simulink model "smm_gait_control"  (R2018b)
settings: configuration reference "Configuration1khz" (kept outside this file)
InitFcn:
  | addpath('./functions/')
  | addpath('./policies/')
  | control_params
values from neighbouring files (symbols this model uses):
  rest = extract_policy_variables('policies/rest.mat')    [control_params.m]
  run_slow = extract_policy_variables('policies/06_run_reduced.mat')    [control_params.m]
  walk_slow = extract_policy_variables('policies/06_walk.mat')    [control_params.m]
undefined symbols (not defined in the file or in its folder): ctrl, Discrete, initial_dx_estimate, initial_dy_estimate, initial_dz_estimate, initial_z_estimate, sample_time, Time
libraries: simulink x42, ctrlSharedLib x7
(part 4 of 5)

== system smm_gait_control/Behavior/Swing Leg Control Secondary/Back//Front PD (velocity) ==
  Desired Position [rad] [back front] : Inport
  Desired Velocity [rad/s] [back front] : Inport  Port=2
  Desired Acceleration [rad/s^2] [back front] : Inport  Port=3
  Measured Position [rad] [back front] : Inport  Port=4
  Measured Velocity [rad/s] [back front] : Inport  Port=5
  Back / Front PositionTracking : Scope  NumInputPorts=2
  Back / Front Velocity Tracking : Scope  NumInputPorts=2
  Feedback / Feedforward : Scope  NumInputPorts=2
  Feedforward Gain : Gain
  Kp_SEA_Trajectory : Constant  Value=ctrl.kp_velocity_swing
  Mux{1..2,12..13} (4 alike) : Mux  Inputs=2
  Product1 : Product
  Selector{,1..3} (4 alike) : Selector  InputPortWidth=2  IndexOptions=Index vector (dialog)  Indices=[1]  OutputSizes=1
  Selector{4..5,7..8} (4 alike) : Selector  InputPortWidth=2  IndexOptions=Index vector (dialog)  Indices=[2]  OutputSizes=1
  Sum7 : Sum  Inputs=|+-
  Sum9 : Sum
  Terminator : Terminator
  Commanded Velocity [rad/s] [back front] : Outport
  wires:
  Kp_SEA_Trajectory/1 -> Product1/2
  Sum9/1 -> Commanded Velocity [rad/s] [back front]/1
  Measured Position [rad] [back front]/1 -> Selector4/1, Selector/1, Sum7/2
  Sum7/1 -> Product1/1
  Product1/1 -> Feedback / Feedforward/1, Sum9/1
  Mux13/1 -> Back / Front PositionTracking/1
  Desired Position [rad] [back front]/1 -> Selector5/1, Selector1/1, Sum7/1
  Mux2/1 -> Back / Front PositionTracking/2
  Selector/1 -> Mux13/1
  Selector1/1 -> Mux13/2
  Selector5/1 -> Mux2/2
  Selector4/1 -> Mux2/1
  Desired Velocity [rad/s] [back front]/1 -> Feedforward Gain/1, Selector8/1, Selector3/1
  Feedforward Gain/1 -> Feedback / Feedforward/2, Sum9/2
  Desired Acceleration [rad/s^2] [back front]/1 -> Terminator/1
  Measured Velocity [rad/s] [back front]/1 -> Selector7/1, Selector2/1
  Mux1/1 -> Back / Front Velocity Tracking/1
  Selector2/1 -> Mux1/1
  Selector7/1 -> Mux12/1
  Mux12/1 -> Back / Front Velocity Tracking/2
  Selector8/1 -> Mux12/2
  Selector3/1 -> Mux1/2

== system smm_gait_control/Behavior/Swing Leg Control Secondary/Lateral PD (torque) ==
  note: (Approximation)
      | This is the lateral torque generated due to the relative
      | acceleration of the motor around the pelvis. Only
      | approximate vertical components are used in the
      | calculation. The lateral components are small.
  Desired Position [rad] : Inport
  Desired Velocity [rad/s] : Inport  Port=2
  Desired Acceleration [rad/s^2] : Inport  Port=3
  Measured Position [rad] : Inport  Port=4
  Measured Velocity [rad/s] : Inport  Port=5
  CoM Z Acceleration [m/s^2] : Inport  Port=6
  Feedback / Feedforward : Scope  NumInputPorts=2
  Kp_SEA_Trajectory : Constant  Value=ctrl.kp_lateral_swing
  Kp_SEA_Trajectory1 : Constant  Value=ctrl.kd_lateral_swing
  Kp_SEA_Trajectory2 : Constant  Value=ctrl.i_lateral_about_pelvis
  Kp_SEA_Trajectory3 : Constant  Value=ctrl.lateral_offset
  Kp_SEA_Trajectory4 : Constant  Value=(ctrl.m_leg_motor + ctrl.m_leg)
  Kp_SEA_Trajectory5 : Constant  Value=-ctrl.g
  Mux13 : Mux  Inputs=2
  Mux2 : Mux  Inputs=2
  Position / Velocity Tracking : Scope  NumInputPorts=2
  Product1 : Product
  Product2 : Product
  Product3 : Product
  Product4 : Product  Inputs=3
  Sum1 : Sum  Inputs=|+-
  Sum2 : Sum  Inputs=|++
  Sum3 : Sum  Inputs=|++
  Sum4 : Sum  Inputs=|+-
  Sum7 : Sum  Inputs=|+-
  Sum9 : Sum  Inputs=++|
  Commanded Torque [Nm] : Outport
  wires:
  Sum3/1 -> Sum2/2, Feedback / Feedforward/2
  Kp_SEA_Trajectory2/1 -> Product3/1
  Desired Acceleration [rad/s^2]/1 -> Product3/2
  Sum2/1 -> Commanded Torque [Nm]/1
  Sum9/1 -> Sum2/1, Feedback / Feedforward/1
  Kp_SEA_Trajectory1/1 -> Product2/2
  Sum1/1 -> Product2/1
  Kp_SEA_Trajectory/1 -> Product1/2
  Measured Position [rad]/1 -> Mux13/1, Sum7/2
  Sum7/1 -> Product1/1
  Product1/1 -> Sum9/1
  Mux13/1 -> Position / Velocity Tracking/1
  Desired Position [rad]/1 -> Mux13/2, Sum7/1
  Mux2/1 -> Position / Velocity Tracking/2
  Desired Velocity [rad/s]/1 -> Mux2/2, Sum1/1
  Product2/1 -> Sum9/2
  Measured Velocity [rad/s]/1 -> Mux2/1, Sum1/2
  Product3/1 -> Sum3/1
  Product4/1 -> Sum3/2
  Kp_SEA_Trajectory4/1 -> Product4/3
  Kp_SEA_Trajectory3/1 -> Product4/2
  Kp_SEA_Trajectory5/1 -> Sum4/1
  CoM Z Acceleration [m/s^2]/1 -> Sum4/2
  Sum4/1 -> Product4/1

== system smm_gait_control/Behavior/Tranform Sensor Measurements to CoM Acceleration Measurement/Compute Body Frame Accelerations ==
  imu accelerations x3 : Inport
  IMU Accel Unfiltered vs Filtered : Scope  NumInputPorts=3
  IMU Two Pole Filter2 : DiscreteTransferFcn  Numerator=[ctrl.A_lpf_accelerometer 0 0]  Denominator=[1 ctrl.B1_lpf_accelerometer ctrl.B2_lpf_accelerometer]  SampleTime=sample_time
  Mux : Mux  Inputs=2
  Selector : Selector  InputPortWidth=6  IndexOptions=Index vector (dialog)  Indices=[1 4]  OutputSizes=1
  Selector1 : Selector  InputPortWidth=6  IndexOptions=Index vector (dialog)  Indices=[2 5]  OutputSizes=1
  Selector2 : Selector  InputPortWidth=6  IndexOptions=Index vector (dialog)  Indices=[3 6]  OutputSizes=1
  accelerations [m/s^2] x3 : Outport
  wires:
  Mux/1 -> Selector/1, Selector2/1, Selector1/1
  imu accelerations x3/1 -> IMU Two Pole Filter2/1, Mux/1
  Selector/1 -> IMU Accel Unfiltered vs Filtered/1
  Selector1/1 -> IMU Accel Unfiltered vs Filtered/2
  Selector2/1 -> IMU Accel Unfiltered vs Filtered/3
  IMU Two Pole Filter2/1 -> Mux/2, accelerations [m/s^2] x3/1

== system smm_gait_control/Behavior/Tranform Sensor Measurements to CoM Acceleration Measurement/Estimate Angular Accelerations2 ==
  Angular Velocities [rad/s] x3 : Inport
  Enabled : Inport  Port=2
  Detect Change : simulink/Logic and Bit Operations/Detect Change  vinit=0  OutDataTypeStr=boolean
  Difference : simulink/Discrete/Difference  ICPrevInput=0.0  OutMin=[]  OutMax=[]  OutDataType=fixdt(1, 16)  OutScaling=2^-10  DoSatur=off
  Gain : Gain  Gain=1/sample_time
  IMU Two Pole Filter : DiscreteTransferFcn  Numerator=[ctrl.A_imu 0 0]  Denominator=[1 ctrl.B1_imu ctrl.B2_imu]  SampleTime=sample_time
  Logical Operator5 : Logic  Operator=NOT  AllPortsSameDT=off  OutDataTypeStr=boolean
  Product : Product
  Angular Accelerations [rad/s^2] x3 : Outport
  wires:
  Detect Change/1 -> Logical Operator5/1
  Difference/1 -> Gain/1
  Gain/1 -> Product/1
  Angular Velocities [rad/s] x3/1 -> Difference/1
  Logical Operator5/1 -> Product/2
  Enabled/1 -> Detect Change/1
  Product/1 -> IMU Two Pole Filter/1
  IMU Two Pole Filter/1 -> Angular Accelerations [rad/s^2] x3/1

== system smm_gait_control/Behavior/Tranform Sensor Measurements to CoM Acceleration Measurement/Estimate Angular Accelerations3 ==
  Angular Velocities [rad/s] x2 : Inport
  Enabled : Inport  Port=2
  Detect Change : simulink/Logic and Bit Operations/Detect Change  vinit=0  OutDataTypeStr=boolean
  Difference : simulink/Discrete/Difference  ICPrevInput=0.0  OutMin=[]  OutMax=[]  OutDataType=fixdt(1, 16)  OutScaling=2^-10  DoSatur=off
  Gain : Gain  Gain=1/sample_time
  IMU Two Pole Filter : DiscreteTransferFcn  Numerator=[ctrl.A_lpf_lateral_accel 0 0]  Denominator=[1 ctrl.B1_lpf_lateral_accel ctrl.B2_lpf_lateral_accel]  SampleTime=sample_time
  Logical Operator5 : Logic  Operator=NOT  AllPortsSameDT=off  OutDataTypeStr=boolean
  Product : Product
  Angular Accelerations [rad/s^2] x2 : Outport
  wires:
  Enabled/1 -> Detect Change/1
  Logical Operator5/1 -> Product/2
  Angular Velocities [rad/s] x2/1 -> Difference/1
  Gain/1 -> Product/1
  Difference/1 -> Gain/1
  Detect Change/1 -> Logical Operator5/1
  Product/1 -> IMU Two Pole Filter/1
  IMU Two Pole Filter/1 -> Angular Accelerations [rad/s^2] x2/1

== system smm_gait_control/Behavior/Filtering/Kalman Filtering/Subsystem ==
  right : Inport
  right? : Inport  Port=2
  left : Inport  Port=3
  Switch : Switch  Criteria=u2 ~= 0
  out : Outport
  wires:
  right/1 -> Switch/1
  right?/1 -> Switch/2
  left/1 -> Switch/3
  Switch/1 -> out/1

== system smm_gait_control/Behavior/Filtering/Kalman Filtering/Subsystem1 ==
  right : Inport
  right? : Inport  Port=2
  left : Inport  Port=3
  Switch : Switch  Criteria=u2 ~= 0
  out : Outport
  wires:
  right/1 -> Switch/1
  right?/1 -> Switch/2
  left/1 -> Switch/3
  Switch/1 -> out/1

== system smm_gait_control/Behavior/Filtering/Kalman Filtering/Subsystem2 ==
  right : Inport
  right? : Inport  Port=2
  left : Inport  Port=3
  Switch : Switch  Criteria=u2 ~= 0
  out : Outport
  wires:
  right/1 -> Switch/1
  right?/1 -> Switch/2
  left/1 -> Switch/3
  Switch/1 -> out/1

== system smm_gait_control/Behavior/Motion Planner/Motion Plan with Simplified Model/Toggle Section Number ==
  1 : Inport
  2 : Inport  Port=2
  3 : Inport  Port=3
  Enable : EnablePort
  Cast : DataTypeConversion  OutDataTypeStr=uint8
  Cast1 : DataTypeConversion  OutDataTypeStr=uint8
  Cast2 : DataTypeConversion  OutDataTypeStr=uint8
  Gain : Gain
  Gain1 : Gain  Gain=2
  Gain2 : Gain  Gain=3
  Max : MinMax  Function=max  Inputs=3
  Out : Outport  InitialOutput=1
  wires:
  Gain/1 -> Cast/1
  Gain1/1 -> Cast1/1
  Gain2/1 -> Cast2/1
  Max/1 -> Out/1
  1/1 -> Gain/1
  2/1 -> Gain1/1
  3/1 -> Gain2/1
  Cast1/1 -> Max/2
  Cast2/1 -> Max/3
  Cast/1 -> Max/1

== matlab function smm_gait_control/Behavior/Swing Leg Control Secondary/Avoid Hitting Mechanical Limits ==
  data: back_cmd output double; front_cmd output double; dback_cmd output double; dfront_cmd output double; ddback_cmd output double; ddfront_cmd output double; back_desired input; dback_desired input; ddback_desired input; front_desired input; dfront_desired input; ddfront_desired input; ctrl parameter
%% Avoid fourbar limits by saturating the commands and ensuring we don't command velocities or 
% accelerations that would push us into the limits when nearby
function [back_cmd, front_cmd, dback_cmd, dfront_cmd, ddback_cmd, ddfront_cmd] ...
    = AvoidFourbarLimits(back_desired,dback_desired, ddback_desired, ...
          front_desired, dfront_desired, ddfront_desired, ...
          ctrl)
    [back_cmd, front_cmd, dback_cmd, dfront_cmd, ddback_cmd, ddfront_cmd] = ...
      AvoidFourbarLimits(back_desired, dback_desired, ddback_desired, ...
                         front_desired, dfront_desired, ddfront_desired, ...
                         ctrl.min_front_bar_angle, ctrl.max_front_bar_angle, ...
                         ctrl.min_back_bar_angle, ctrl.max_back_bar_angle);
end

== matlab function smm_gait_control/Behavior/Select Gait Number ==
  data: system_time input; gait_id output; step_number input; enable_locomotion output; at_rest input; disable_locomotion output
function [gait_id, enable_locomotion, disable_locomotion] = select_gait(system_time, step_number, at_rest)

  if system_time < 5
    gait_id = 1;
    enable_locomotion = false;
    disable_locomotion = true;
  else
    enable_locomotion = true;
    disable_locomotion = false;
    if step_number <= 10
      gait_id = 2;
    elseif step_number > 10 && step_number <= 20
      gait_id = 3;
    elseif step_number > 20 && step_number <= 30
      gait_id = 4;
    elseif step_number > 30 && step_number <= 40
      gait_id = 3;
    elseif step_number > 40 && step_number <= 50
      gait_id = 2;
    else
      gait_id = 1;
      if at_rest
        enable_locomotion = false;
        disable_locomotion = true;
      end
    end
  end
      
end

== matlab function smm_gait_control/Behavior/2D Lateral Stance Control2 ==
  data: F_leg input; lateral_torque output; ctrl parameter
function lateral_torque = lateral_stance_control_on_boom(F_leg,ctrl)
    lateral_torque = F_leg*ctrl.lateral_offset*(ctrl.m_total-(ctrl.m_leg_motor+ctrl.m_leg))/ctrl.m_total;
end

== stateflow chart smm_gait_control/Behavior/Contact State Machine/Left Leg State ==
  state Stance
  state Twilight
  state Swing
  (junction 196) -> Stance
  (junction 198) -> (junction 196)
  Stance -> Twilight : [terminate_contact && force < touchdown_threshold]
  Twilight -> Swing : after(ctrl.twilight_time, sec)
  (default) -> Swing
  Swing -> (junction 198) : [force > touchdown_threshold]
  data: force input; touchdown_threshold input; ctrl parameter; Stance output boolean; Twilight output boolean; Swing output boolean; terminate_contact input

== matlab function smm_gait_control/Behavior/2D Lateral Stance Control3 ==
  data: F_leg input; lateral_torque output; ctrl parameter
function lateral_torque = lateral_stance_control_on_boom(F_leg,ctrl)
    lateral_torque = F_leg*ctrl.lateral_offset*(ctrl.m_total-(ctrl.m_leg_motor+ctrl.m_leg))/ctrl.m_total;
end

== matlab function smm_gait_control/Behavior/Centroidal Model Control/Stance Control ==
  data: enable input; x_state_desired output; z_state_desired output; feedforward_term_1 output; feedforward_term_2 output; feedforward_term_3 output; feedback_term_1 output; feedback_term_2 output; feedback_term_3 output; reference input size=[6 1]; K_lqr input size=[3 6]; feedforward_terms input size=[3 1]; phase input; x_state_1 input; x_state_2 input; Fx1 output; z_state input; theta_state input; leg_length_primary input; leg_length_secondary input; Fz_disturbance input; right_is_primary input; plan_not_ready input; Fz1 output; Fx2 output; Fz2 output; ctrl parameter
%% Create motion plans for the centroidal model
% state = [x, dx/dt, z, dz/dt, theta, dtheta/dt]
% F_single_support = [Fx, Fz]
% F_double_support = [Fx, Fz1, Fz2]
function [ x_state_desired, z_state_desired, ...
           feedforward_term_1, feedforward_term_2, feedforward_term_3, ...
           feedback_term_1, feedback_term_2, feedback_term_3, ...
           Fx1, Fz1, Fx2, Fz2] = ...
           centroidal_control(enable, reference, K_lqr, feedforward_terms, ...
                              phase, x_state_1, x_state_2, z_state, theta_state, ...
                              leg_length_primary, leg_length_secondary, Fz_disturbance, right_is_primary, plan_not_ready, ctrl)

  persistent p_prev_x_state_desired p_prev_z_state_desired p_prev_fx1 p_prev_fx2 p_prev_fz1 p_prev_fz2
  if isempty(p_prev_x_state_desired)
    p_prev_x_state_desired = [0; 0]; 
    p_prev_z_state_desired = [0; 0];
    p_prev_fx1 = 0;
    p_prev_fx2 = 0; 
    p_prev_fz1 = 0; 
    p_prev_fz2 = 0;
  end
                            
  % Nothing to be done for flight phase, return
  if phase == 0
    Fx1 = 0;
    Fz1 = 0;
    Fx2 = 0;
    Fz2 = 0;
    x_state_desired = [0; 0];
    z_state_desired = [0; 0];
    feedforward_term_1 = 0;
    feedforward_term_2 = 0;
    feedforward_term_3 = 0;
    feedback_term_1 = 0;
    feedback_term_2 = 0;
    feedback_term_3 = 0;
    p_prev_x_state_desired = [0; 0]; 
    p_prev_z_state_desired = [0; 0];
    p_prev_fx1 = 0;
    p_prev_fx2 = 0; 
    p_prev_fz1 = 0; 
    p_prev_fz2 = 0;
    return;
  end
  
  % Compute feedback control
  error = reference - [x_state_1; z_state; theta_state];
  F_feedback = K_lqr*error;
%   % use neutral feedforward in single support
%   if phase == 1
%     feedforward_terms(2) = acos(min(max(x_state_1(1)/z_state(1),-1),1));
%   end
  % Create control output variables
  input = F_feedback + feedforward_terms; % [Fx, Fz1, Fz2]
  if phase == 1
    F_mag = input(1);
    F_angle = input(2);
    Fx1 = F_mag*cos(F_angle);
    Fz1 = F_mag*sin(F_angle);
    Fz1 = max(Fz1 + Fz_disturbance, 0); % Fz > 0 constraint
    Fz2 = 0;
    Fx1 = max(min(Fx1, 0.5*Fz1), -0.5*Fz1); % saturate to friction cone
    Fx2 = 0;
  else % phase == 2, double support
    Fz1 = input(2);
    Fz2 = input(3);
    Fz1 = max(Fz1 + Fz_disturbance*Fz1/(Fz1+Fz2+eps),0); % Fz > 0 constraint
    Fz2 = max(Fz2 + Fz_disturbance*Fz2/(Fz1+Fz2+eps),0);
    Fx1 = input(1)*Fz1/(Fz1+Fz2+eps); % distribute x force proportionally to z forces
    Fx2 = input(1)*Fz2/(Fz1+Fz2+eps);
    Fx1 = max(min(Fx1, 0.5*Fz1), -0.5*Fz1); % saturate to friction cone
    Fx2 = max(min(Fx2, 0.5*Fz2), -0.5*Fz2);
  end
  
  % Apply boom compensation to vertical forces
  if right_is_primary
    Fz1 = ctrl.fz_boom_compensation_right * Fz1;
    Fz2 = ctrl.fz_boom_compensation_left * Fz2;
  else
    Fz1 = ctrl.fz_boom_compensation_left * Fz1;
    Fz2 = ctrl.fz_boom_compensation_right * Fz2;
  end
  
%   % Prevent leg hyperextension
%   if leg_length_primary(2) > 0 && leg_length_primary(1) > ctrl.stop_stance_leg_extension
%     %leg_over_extension = (leg_length_primary(1) - ctrl.stop_stance_leg_extension) ...
%     %                     / (ctrl.max_stance_leg_extension - ctrl.stop_stance_leg_extension);
%     %attenuation = exp(-ctrl.hyperextension_attenuation_rate*leg_over_extension);
%     attenuation = 0.2;
%     Fx1 = attenuation * Fx1;
%     Fz1 = attenuation * Fz1;
%   end
%   if leg_length_secondary(2) > 0 && leg_length_secondary(1) > ctrl.max_stance_leg_extension
%     %leg_over_extension = (leg_length_secondary(1) - ctrl.stop_stance_leg_extension) ...
%     %                     / (ctrl.max_stance_leg_extension - ctrl.stop_stance_leg_extension);
%     %attenuation = exp(-ctrl.hyperextension_attenuation_rate*leg_over_extension);
%     attenuation = 0.2;
%     Fx2 = attenuation * Fx2;
%     Fz2 = attenuation * Fz2;
%   end
  
  if phase == 1 || phase == 2
    Fz1 = max(Fz1, 90);
  end
  if phase == 2
    Fz2 = max(Fz2, 90);
  end
  
  % Output desired state
  x_state_desired = reference(1:2);
  z_state_desired = reference(3:4);
  
  % If plan is not ready, just hold previous outputs
  if plan_not_ready
    Fx1 = p_prev_fx1;
    Fx2 = p_prev_fx2;
    Fz1 = p_prev_fz1;
    Fz2 = p_prev_fz2;
    x_state_desired = p_prev_x_state_desired; 
    z_state_desired = p_prev_z_state_desired;
  end
  
  % Output logging variables
  feedforward_term_1 = feedforward_terms(1);
  feedforward_term_2 = feedforward_terms(2);
  feedback_term_1 = F_feedback(1);
  feedback_term_2 = F_feedback(2);
  if phase == 2
    feedforward_term_3 = feedforward_terms(3);
    feedback_term_3 = F_feedback(3);
  else
    feedforward_term_3 = 0;
    feedback_term_3 = 0;
  end
  
  % store previous values
  p_prev_x_state_desired = x_state_desired; 
  p_prev_z_state_desired = z_state_desired;
  p_prev_fx1 = Fx1;
  p_prev_fx2 = Fx2; 
  p_prev_fz1 = Fz1; 
  p_prev_fz2 = Fz2;
  
end

== matlab function smm_gait_control/Behavior/SEA Measurements/Leg Dynamics Right ==
  data: tau_back input; tau_front input; axial_force output; leg_width input; leg_length input; ortho_force output
function [axial_force, ortho_force] = fcn(tau_back, tau_front, leg_width, leg_length)

  % prevent divide by zero
  leg_width(1) = max(leg_width(1),eps);
  leg_length(1) = max(leg_length(1),eps);

  % forces and torques
  hip_torque = tau_front + tau_back;
  spread_torque = tau_front - tau_back;
  axial_force = zeros(2,1);
  axial_force(1) = spread_torque(1) / leg_width(1);
  ortho_force = zeros(2,1);
  ortho_force(1) = hip_torque(1) / leg_length(1);
  
  % time derivatives
  axial_force(2) = (leg_width(1)*spread_torque(2) - spread_torque(1)*leg_width(2)) / (leg_width(1)*leg_width(1));
  ortho_force(2) = (leg_length(1)*hip_torque(2) - hip_torque(1)*leg_length(2)) / (leg_length(1)*leg_length(1));
  
end

== stateflow chart smm_gait_control/Behavior/Contact State Machine/Right Leg State ==
  state Stance
  state Twilight
  state Swing
  (junction 196) -> Stance
  (junction 198) -> (junction 196)
  Stance -> Twilight : [terminate_contact && force < touchdown_threshold]
  Twilight -> Swing : after(ctrl.twilight_time, sec)
  (default) -> Swing
  Swing -> (junction 198) : [force > touchdown_threshold]
  data: force input; touchdown_threshold input; terminate_contact input; ctrl parameter; Stance output boolean; Twilight output boolean; Swing output boolean

== matlab function smm_gait_control/Behavior/Motion Planner/Motion Plan with Simplified Model/Model Predictive Control (LQR) ==
  settings: updateMethod=DISCRETE
  data: replan input boolean size=1; plan_length input double size=1; time_plan input double size=[ctrl.max_trajectory_length 1]; K_lqr_plan output double size=[ctrl.max_trajectory_length 3 6]; feedforward_plan output double size=[ctrl.max_trajectory_length 3]; state_plan input double size=[ctrl.max_trajectory_length 6]; accel_plan input double size=[ctrl.max_trajectory_length 2]; phase input double size=1; x_state_1 input double size=2; x_state_2 input double size=2; z_state input double size=2; theta_state input double size=2; rest_length input double size=1; ctrl parameter size=1
%% Compute finite horizon LQR for single support or double support phases
% Single support actions = [F_magnitude, F_angle]
% Double support actions = [Fx, Fz1, Fz2]
function [ K_lqr_plan, feedforward_plan ] = ...
           motion_planner(replan, plan_length, time_plan, state_plan, accel_plan, ...
                          phase, x_state_1, x_state_2, z_state, theta_state, rest_length, ctrl)
               
  % Specify variable sizes for Simulink coder (must be edited if max trajectory length is changed)
  coder.varsize('p_feedforward_plan',[101, 3]);
  coder.varsize('p_K_lqr_plan',[101, 3, 6]);

  % Declare persistent variables for plans
  persistent p_K_lqr_plan p_feedforward_plan
  if isempty(p_K_lqr_plan) || phase == 0
    p_K_lqr_plan = zeros(1,3,6);
    p_feedforward_plan = zeros(1,3);
  end

  % SINGLE/DOUBLE SUPPORT: Calculate finite horizon LQR feedback/feedforward
  if replan && (phase == 1 || phase == 2)
    % Generate feedforward control for the trajectory
    d_feet = x_state_2(1) - x_state_1(1);
    p_feedforward_plan = compute_feedforward(phase, state_plan(1:plan_length,1), state_plan(1:plan_length,3), ...
                                             accel_plan(1:plan_length,1), accel_plan(1:plan_length,2), ...
                                             ctrl.m_total, ctrl.g, rest_length, d_feet);
    % Compute optimal finite horizon LQR gains for the plan
    p_K_lqr_plan = zeros(plan_length, 3, 6);
    if phase == 1 % single support
      P_lqr = ctrl.H_lqr_single;
      R = ctrl.R_lqr_single;
      Q = ctrl.Q_lqr_single;
    else % double support
      P_lqr = ctrl.H_lqr_double;
      R = ctrl.R_lqr_double;
      Q = ctrl.Q_lqr_double;
    end
    for i = plan_length-1:-1:1
        dt = time_plan(i+1) - time_plan(i);
        x_ref = state_plan(i,1);
        z_ref = state_plan(i,3);
        if phase == 1 % single support
          % (F_mag, F_angle) space
          F_mag_ref = p_feedforward_plan(i,1);
          F_angle_ref = p_feedforward_plan(i,2);
          A_single = A_centroidal_linearized_single(F_mag_ref, F_angle_ref, dt, ctrl.i_robot);
          B_single = B_centroidal_linearized_single(F_mag_ref, F_angle_ref, x_ref, z_ref, dt, ctrl.i_robot, ctrl.m_total);
          p_K_lqr_plan(i,1:2,:) = (R + B_single'*P_lqr*B_single) \ (B_single'*P_lqr*A_single);
          P_lqr = Q + A_single'*P_lqr*A_single ...
                  - (A_single'*P_lqr*B_single) * ((R + B_single'*P_lqr*B_single) \ (B_single'*P_lqr*A_single));
        else % phase == 2, double support
          Fx_ref = p_feedforward_plan(i,1);
          Fz_ref = sum(p_feedforward_plan(i,2:3),2); % sum 2 vertical forces
          A_double = A_centroidal_linearized(Fx_ref, Fz_ref, dt, ctrl.i_robot);
          B_double = B_centroidal_linearized_double(x_ref, z_ref, dt, ctrl.i_robot, ctrl.m_total, d_feet);
          p_K_lqr_plan(i,1:3,:) = (R + B_double'*P_lqr*B_double) \ (B_double'*P_lqr*A_double);
          P_lqr = Q + A_double'*P_lqr*A_double ...
                  - (A_double'*P_lqr*B_double) * ((R + B_double'*P_lqr*B_double) \ (B_double'*P_lqr*A_double));
        end
    end
  end
  
  % Output persistent variables
  K_lqr_plan = zeros(101,3,6);
  feedforward_plan = zeros(101,3);
  output_length = size(p_feedforward_plan,1);
  K_lqr_plan(1:output_length,:,:) = p_K_lqr_plan;
  feedforward_plan(1:output_length,:) = p_feedforward_plan;
  
%   n = size(time_plan,1);
%   feedforward_plan = repmat([ctrl.m_total*ctrl.g, pi/2], n, 1);
%   K_lqr_plan = zeros(1,3,6);
  
end

%% Linearlized dynamics matrices
function [A] = A_centroidal_linearized(Fx_total, Fz_total, dt, I) 
 A = [1, dt, 0, 0,  0, 0; ...
      0,  1, 0, 0,  0, 0; ...
      0,  0, 1, dt, 0, 0; ...
      0,  0, 0,  1, 0, 0; ...
      0,  0, 0,  0, 1, dt; ...
      Fz_total*dt/I, 0, -Fx_total*dt/I, 0, 0, 1];
end

function [B] = B_centroidal_linearized_double(x, z, dt, I, m, d) 
 B = [0,       0,          0; ...
      dt/m,    0,          0; ...
      0,       0,          0; ...
      0,       dt/m,       dt/m; ...
      0,       0,          0; ...
      -z*dt/I, x*dt/I,    (x+d)*dt/I];         
end

function [A] = A_centroidal_linearized_single(F_mag, F_angle, dt, I) 
 A = [1, dt, 0, 0,  0, 0; ...
      0,  1, 0, 0,  0, 0; ...
      0,  0, 1, dt, 0, 0; ...
      0,  0, 0,  1, 0, 0; ...
      0,  0, 0,  0, 1, dt; ...
      F_mag*sin(F_angle)*dt/I, 0, -F_mag*cos(F_angle)*dt/I, 0, 0, 1];
end

function [B] = B_centroidal_linearized_single(F_mag, F_angle, x, z, dt, I, m) 
 B = [0,       0; ...
      (dt/m)*cos(F_angle),    -(dt/m)*F_mag*sin(F_angle); ...
      0,       0; ...
      (dt/m)*sin(F_angle),     (dt/m)*F_mag*cos(F_angle); ...
      0,       0; ...
      (dt/I)*(-z*cos(F_angle)+x*sin(F_angle)), (dt/I)*(z*F_mag*sin(F_angle)+x*F_mag*cos(F_angle))];         
end

%% Calculates feedforward forces (assumes reference ddtheta/ddt = 0)
function [F_feedforward] = compute_feedforward( phase, x_pos, z_pos, x_accel, z_accel, m, g, l0, d_feet)
  if phase == 1 % Single support: Point GRF through CoM
    % (F_mag, F_angle) space
    F_angle = acos(min(max(x_pos./z_pos,-1),1));
    %F_mag = m*sqrt((0*x_accel).^2 + (z_accel+g).^2); % only use Z accel
    F_mag = m*sqrt((x_accel).^2 + (z_accel+g).^2);
    F_feedforward = [F_mag, F_angle, zeros(size(F_mag))];
  elseif phase == 2 % Double support: ???
    % If we exactly solve for desired accelerations ...
    %   Fx = m*x_accel;
    %   Fz1 = m*(z_accel + g + (x_pos.*z_accel - z_pos.*x_accel + g*x_pos)/d_feet); % -I/d*theta_accel = 0
    %   Fz2 = m*(z_pos.*x_accel - x_pos.*z_accel - g*x_pos)/d_feet; % +I/d*theta_accel = 0
    % Or if we put the net force vector through the CoM and scale z forces to leg compression ...
    Fz_total = m*(z_accel + g);
    leg_compress_1 = max(l0 - sqrt(x_pos.^2 + z_pos.^2), 0);
    leg_compress_2 = max(l0 - sqrt((x_pos + d_feet).^2 + z_pos.^2), 0);
    Fz1 = Fz_total.*leg_compress_1./(leg_compress_1 + leg_compress_2 + eps);
    Fz2 = Fz_total.*leg_compress_2./(leg_compress_1 + leg_compress_2 + eps);
    Fx = (x_pos.*Fz1 + (x_pos + d_feet).*Fz2) ./ z_pos;
    F_feedforward = [Fx, Fz1, Fz2];
  else
    F_feedforward = zeros(size(x_pos,1),3);
  end
end

== matlab function smm_gait_control/Behavior/Motion Planner/Motion Plan with Simplified Model/Plan Simplified Model ==
  settings: updateMethod=DISCRETE
  data: plan_length output double size=1; enable input; time_plan output double size=[ctrl.max_trajectory_length 1]; state_plan output double size=[ctrl.max_trajectory_length 6]; accel_plan output double size=[ctrl.max_trajectory_length 2]; replan input; section input uint8; entered_double_support input; t_plan input; x_state_1 input; x_state_2 input; z_state input; theta_state input; grf_xz_primary input; prev_phase input; delayed_state input; gait_id input; rest parameter; angle_of_attack output double size=1; double_support_start_time output double size=1; double_support output boolean size=1; run_slow parameter; walk_slow parameter; ctrl parameter; plan_end_time output double size=1; rest_length output double size=1; takeoff_leg output double size=1; neutral_point output double size=1; k_placement output double size=1
%% Create motion plans for the centroidal model
% Flight: Not applicable
% Single support: CoM plan until takeoff or initial single support
% Double support: CoM plan until takeoff (initial single support)
%
% section = 1:flight apex, 2:single init, 3:single apex
% state = [x, dx/dt, z, dz/dt, theta, dtheta/dt]
%
% (Code using specific gait structs is repeated due to Simulink limitations)
% (tip: if out of stack space, pass by reference, [outputs, struct] = fcn(inputs, struct) )
function [ plan_length, time_plan, state_plan, accel_plan, angle_of_attack, double_support_start_time, double_support, plan_end_time, rest_length, takeoff_leg, neutral_point, k_placement ] = ...
           motion_planner(enable, replan, section, entered_double_support, t_plan, ...
                          x_state_1, x_state_2, z_state, theta_state, grf_xz_primary, prev_phase, delayed_state, ...
                          gait_id, rest, run_slow, walk_slow, ctrl)
  % Compiler runs out of heap space (C1060) when passing in too many policies

  % Specify variable sizes for Simulink coder (must be edited if max trajectory length is changed)
  coder.varsize('p_time_plan',101);
  coder.varsize('p_state_plan',[101, 6]);
  coder.varsize('p_accel_plan',[101, 2]);
  
  % Declare persistent variables for plans
  persistent p_time_plan p_state_plan p_accel_plan p_angle_of_attack p_double_support_start_time p_double_support p_takeoff_leg p_neutral_point p_k_placement
  if isempty(p_time_plan) 
    p_time_plan = zeros(1,1);
    p_state_plan = zeros(1,6);
    p_accel_plan = zeros(1,2);
    p_angle_of_attack = zeros(1,1);
    p_double_support_start_time = zeros(1,1);
    p_double_support = false;
    p_takeoff_leg = 1;
    p_neutral_point = 0;
    p_k_placement = 0;
  end
  
  % FLIGHT: Look up the next angle of attack
  if replan && section == 1
    if enable % If enabled, find touchdown angle from lookup table
      state = [x_state_1; z_state]';
      % Select a gait
      switch(gait_id)
        case 1
          p_angle_of_attack = FindTouchdownAngle(state, section, rest);
        case 2
          p_angle_of_attack = FindTouchdownAngle(state, section, walk_slow);
        case 3
          p_angle_of_attack = FindTouchdownAngle(state, section, run_slow);
      end
    else      % Otherwise point leg down (could replace with heuristic control)
      p_angle_of_attack = 90;
    end
  end

  % SINGLE SUPPORT: Look up CoM motion plan and angle of attack (if applicable)
  if replan && (section == 2 || section == 3)
    if enable  % If enabled, generate a CoM motion plan from the simplified model
      state = [x_state_1; z_state]';
      switch(gait_id)
        case 1
          [ p_state_plan, p_accel_plan, p_time_plan, p_angle_of_attack, p_double_support_start_time, p_double_support, p_takeoff_leg, p_neutral_point, p_k_placement ] ...
            = FindOfflineComPlanInternal( state, section, prev_phase, delayed_state, rest);
        case 2
          [ p_state_plan, p_accel_plan, p_time_plan, p_angle_of_attack, p_double_support_start_time, p_double_support, p_takeoff_leg, p_neutral_point, p_k_placement ] ...
            = FindOfflineComPlanInternal( state, section, prev_phase, delayed_state, walk_slow);
        case 3
          [ p_state_plan, p_accel_plan, p_time_plan, p_angle_of_attack, p_double_support_start_time, p_double_support, p_takeoff_leg, p_neutral_point, p_k_placement ] ...
            = FindOfflineComPlanInternal( state, section, prev_phase, delayed_state, run_slow);
      end
      p_state_plan = [p_state_plan, ...  % include trajectory for torso pitch
                      repmat([ctrl.desired_torso_pitch,0],length(p_time_plan),1)];    
    else       % Otherwise, generate static reference trajectory
      t_end = ctrl.max_lqr_horizon;
      p_time_plan = (0:ctrl.dt_lqr:t_end)';
      n_points = length(p_time_plan);
      p_accel_plan = zeros(n_points, 2);
      p_double_support_start_time = 0.300;
      p_takeoff_leg = 1;
      % target double support at rest, single support otherwise
      if gait_id == 1
        % double support static
        p_double_support = true;
        x_steady_target = 0.5 * (x_state_1(1) + sign(x_state_1(1)) * abs(ctrl.static_double_x_pos_stance));
        p_state_plan = repmat([x_steady_target, 0, ctrl.static_double_z_pos_stance, 0, 0, 0], n_points, 1);
      else
        % single support static
        p_double_support = false;
        x_steady_target = ctrl.static_single_x_pos_stance;
        p_state_plan = repmat([x_steady_target, 0, ctrl.static_single_z_pos_stance, 0, 0, 0], n_points, 1);
      end
   end
  end
  
  % Update plan to steady state if entering double support with disabled locomotion
  if entered_double_support && ~enable
    n_points = length(p_time_plan);
    d_feet = x_state_2(1) - x_state_1(1);
    x_steady_target = -0.5 * d_feet;
    p_state_plan = repmat([x_steady_target, 0, ctrl.static_double_z_pos_stance, 0, 0, 0], n_points, 1);
  end
  
  % Truncate stored motion plan when entering double support
  if entered_double_support && enable && ~replan
%     end_time = p_time_plan(end);
%     if t_plan > end_time
%       p_time_plan = (end_time:ctrl.dt_lqr:(end_time+0.050))';
%       p_double_support_start_time = p_time_plan(end);
%       p_state_plan = repmat(p_state_plan(end,:),numel(p_time_plan),1);
%       p_accel_plan = zeros(numel(p_time_plan),2);
%     else
%       init_state = interp1(p_time_plan, p_state_plan, t_plan,'linear');
%       init_accel = interp1(p_time_plan, p_accel_plan, t_plan,'linear');
%       select_remaining = p_time_plan - t_plan > 0; 
%       p_time_plan = [t_plan; p_time_plan(select_remaining, :)];
%       p_state_plan = [init_state; p_state_plan(select_remaining,:)];
%       p_accel_plan = [init_accel; p_accel_plan(select_remaining,:)];
%     end

    %init_state = interp1(p_time_plan, p_state_plan, p_double_support_start_time,'linear');
    %init_accel = interp1(p_time_plan, p_accel_plan, p_double_support_start_time,'linear');
    if p_double_support
      select_remaining = p_time_plan >= p_double_support_start_time; 
    else % unintentional double support, truncate plan approximately
      select_remaining = p_time_plan >= t_plan - 0.010; 
    end
    % edge case: entered double support, but nothing left in plan, hold last two points
    if ~any(select_remaining)
      select_remaining(end-1:end) = true;
    end
    p_time_plan = p_time_plan(select_remaining, :);
    p_state_plan = p_state_plan(select_remaining,:);
    p_accel_plan = p_accel_plan(select_remaining,:);
    
  end
  
  % Output persistent variables
  time_plan = zeros(101,1);
  state_plan = zeros(101,6);
  accel_plan = zeros(101,2);
  plan_length = numel(p_time_plan);
  time_plan(1:plan_length) = p_time_plan;
  state_plan(1:plan_length,:) = p_state_plan;
  accel_plan(1:plan_length,:) = p_accel_plan;
  angle_of_attack = p_angle_of_attack;
  double_support_start_time = p_double_support_start_time;
  double_support = p_double_support;
  takeoff_leg =  p_takeoff_leg;
  plan_end_time = p_time_plan(end);
  neutral_point = p_neutral_point;
  k_placement = p_k_placement;
 
  % Output current model rest length
  switch(gait_id)
    case 1
      rest_length = rest.model.l0;
    case 2
      rest_length = walk_slow.model.l0;
    case 3
      rest_length = run_slow.model.l0;
    otherwise
      rest_length = 1.1;
  end
  
end


%% Lookup motion plan for the CoM at a single support Poincare section
% state = [x, dx/dt, z, dz/dt]
% to_double_support = true if leg will touchdown, false otherwise
function [ state_plan, accel_plan, time_plan, angle_of_attack, touchdown_time, to_double_support, takeoff_leg, neutral_point, k_placement] = ...
          FindOfflineComPlanInternal( initial_state, initial_section, prev_phase, delayed_state, policy)
%  coder.inline('never');
  % Initialize some outputs
  neutral_point = 0;
  k_placement = 0;
  takeoff_leg = 1; % Takeoff primary leg (if taking off)
  % Nothing to be done for flight apex Poincare section
  if initial_section == 1
    state_plan = zeros(1,4);
    accel_plan = zeros(1,2);
    time_plan = zeros(1,1);
    angle_of_attack = FindTouchdownAngle(initial_state, initial_section, policy);
    touchdown_time = 0;
    to_double_support = false;
    return;
  end
  persistent p_neutral_point
  if isempty(p_neutral_point)
    p_neutral_point = 0;
  end
  % Look up closest valid trajectory
 closest_bin_idx = FindClosestBinIdx(initial_state, initial_section, policy);
  % Find state and accel plans
  if initial_section == 2 % SSI
    %closest_bin_idx = 20756;
    % Use valid point mapping to override invalid points
    closest_bin_idx = policy.com_traj.ssi.valid_map(closest_bin_idx);
    % Use directory to lookup where trajectory is stored
    location = policy.com_traj.ssi.directory(closest_bin_idx,:);
    % Find timings
    time_plan = double(policy.com_traj.ssi.timings(location(1):location(2))');
    % Concatenate state and accel plans
    state_plan = double([ policy.com_traj.ssi.x_pos(location(1):location(2))', ...
                           policy.com_traj.ssi.x_vel(location(1):location(2))', ...
                           policy.com_traj.ssi.z_pos(location(1):location(2))', ...
                           policy.com_traj.ssi.z_vel(location(1):location(2))' ]);
    accel_plan = double([ policy.com_traj.ssi.x_acc(location(1):location(2))', ...
                          policy.com_traj.ssi.z_acc(location(1):location(2))' ]);
    to_double_support = policy.com_traj.ssi.to_double_support(closest_bin_idx);
    % Lookup touchdown time and angle if planning a double support phase
    if to_double_support
      closest_final_bin_idx = FindClosestBinIdx(state_plan(end,:), 3, policy);
      closest_final_bin_idx = policy.com_traj.ssa.valid_map(closest_final_bin_idx);
      next_double_support_time = policy.com_traj.ssa.touchdown_times(closest_final_bin_idx);
      touchdown_time = time_plan(end) + next_double_support_time;
      angle_of_attack = policy.angle.ssa(closest_final_bin_idx);
      % Use directory to lookup where trajectory is stored
      location = policy.com_traj.ssa.directory(closest_final_bin_idx,:);
      % Find next section timings and x velocity plan
      next_time_plan = double(policy.com_traj.ssa.timings(location(1):location(2))');
      next_x_vel_plan = double(policy.com_traj.ssa.x_vel(location(1):location(2))');
      % Compute linear feedback for leg placement
      com_x_vel_expected = interp1(next_time_plan, next_x_vel_plan, next_double_support_time, 'linear');
      x_target = -policy.model.l0 * cosd(angle_of_attack);
      p_neutral_point = - 0.5 * mean([state_plan(:,2); next_x_vel_plan]) * (time_plan(end) + next_time_plan(end));
      k_placement = ( x_target - p_neutral_point ) / ( policy.desired_x_velocity - com_x_vel_expected );
    else % Entering flight
      touchdown_time = time_plan(end);
      angle_of_attack = FindTouchdownAngle(state_plan(end,:), 1, policy);
      com_x_vel_expected = state_plan(end,2);
      x_target = -policy.model.l0 * cosd(angle_of_attack);
      p_neutral_point = - 0.5 * mean(state_plan(:,2)) * time_plan(end);
      k_placement = ( x_target - p_neutral_point ) / ( policy.desired_x_velocity - com_x_vel_expected );
    end
  else % initial_section == 3, SSA
    %closest_bin_idx = 2624;
    % Use valid point mapping to override invalid points
    closest_bin_idx = policy.com_traj.ssa.valid_map(closest_bin_idx);
    % Use directory to lookup where trajectory is stored
    location = policy.com_traj.ssa.directory(closest_bin_idx,:);
    % Find timings
    time_plan = double(policy.com_traj.ssa.timings(location(1):location(2))');
    % Concatenate state and accel plans
    state_plan = double([ policy.com_traj.ssa.x_pos(location(1):location(2))', ...
                           policy.com_traj.ssa.x_vel(location(1):location(2))', ...
                           policy.com_traj.ssa.z_pos(location(1):location(2))', ...
                           policy.com_traj.ssa.z_vel(location(1):location(2))' ]);
    accel_plan = double([ policy.com_traj.ssa.x_acc(location(1):location(2))', ...
                          policy.com_traj.ssa.z_acc(location(1):location(2))' ]);
    to_double_support = true;
    % Lookup touchdown time and angle if planning a double support phase
    touchdown_time = policy.com_traj.ssa.touchdown_times(closest_bin_idx);
    angle_of_attack = policy.angle.ssa(closest_bin_idx);
    % Compute linear feedback for leg placement
    com_x_vel_expected = interp1(time_plan, state_plan(:,2), touchdown_time, 'linear');
    x_target = -policy.model.l0 * cosd(angle_of_attack);
    k_placement = ( x_target - p_neutral_point ) / ( policy.desired_x_velocity - com_x_vel_expected );
  end
  % Output persistent variables
  neutral_point = p_neutral_point;
  
  % time dilation
  alpha_dilate = 1.10;
  state_plan(:,2) = state_plan(:,2) / alpha_dilate;
  state_plan(:,4) = state_plan(:,4) / alpha_dilate;
  accel_plan = accel_plan / (alpha_dilate^2);
  time_plan = time_plan * alpha_dilate;
  touchdown_time = touchdown_time * alpha_dilate;
end

== matlab function smm_gait_control/Behavior/Swing Leg Control Secondary/Convert CoM (X,Y,Z) to  (Leg Angles, Leg Length) ==
  data: desired_leg_length output; X_star input; Y_star input; Z_star input; right_left input; pelvis2com_pos input; desired_alpha output; desired_beta output; pelvis2com_vel input; roll input; pitch input; sagittal_angle input; lateral_angle input; leg_length input; ctrl parameter
%% Convert Foot2CoM vector from (X, Y, Z) to (leg length, leg angle) space
function [ desired_leg_length, desired_alpha, desired_beta ]  =  ...
          ConvertToJointAnglesAndLegLength(X_star, Y_star, Z_star, right_left,...
                           pelvis2com_pos, pelvis2com_vel, ...
                           roll, pitch, sagittal_angle, lateral_angle, leg_length,...
                           ctrl) 

    q = [roll(1), pitch(1), sagittal_angle(1), lateral_angle(1), leg_length(1)];
    dq = [roll(2), pitch(2), sagittal_angle(2), lateral_angle(2), leg_length(2)];
    [desired_alpha, desired_beta, desired_leg_length] = ...
      ConvertComPositionToLegAnglesAndLegLength(X_star, Y_star, Z_star, right_left, ...
                                                pelvis2com_pos, pelvis2com_vel, ...
                                                q, dq, ctrl.lateral_offset);
    desired_beta = saturate(desired_beta, ctrl.min_lateral_beta, ctrl.max_lateral_beta);
end

function [desired_saturated] = saturate(desired, min_lateral_beta, max_lateral_beta)
    desired_saturated = desired;
    if desired(1) < min_lateral_beta
        desired_saturated = [min_lateral_beta; 0; 0];
    elseif desired(1) > max_lateral_beta
        desired_saturated = [max_lateral_beta; 0; 0];    
    end
end

== matlab function smm_gait_control/Behavior/Primary-Secondary Routing Inputs ==
  data: right_is_primary input size=1; leg_angle_primary output size=2; leg_angle_right input size=2; leg_length_right input size=2; leg_width_right input size=2; leg_roll_right input size=2; back_load_right input size=2; back_motor_right input size=2; front_load_right input size=2; front_motor_right input size=2; lateral_right input size=2; axial_force_right input; grf_xz_right input; foot2com_x_right input; foot2com_z_right input; x_state_right input; leg_angle_left input size=2; leg_length_left input size=2; leg_width_left input size=2; leg_roll_left input size=2; back_load_left input size=2; back_motor_left input size=2; front_load_left input size=2; front_motor_left input size=2; lateral_left input size=2; leg_length_primary output size=2; leg_width_primary output size=2; leg_roll_primary output size=2; back_load_primary output size=2; back_motor_primary output size=2; front_load_primary output size=2; front_motor_primary output size=2; lateral_primary output size=2; axial_force_primary output; grf_xz_primary output; foot2com_x_primary output; foot2com_z_primary output; x_state_primary output; leg_angle_secondary output size=2; leg_length_secondary output size=2; leg_width_secondary output size=2; leg_roll_secondary output size=2; back_load_secondary output size=2; back_motor_secondary output size=2; front_load_secondary output size=2; front_motor_secondary output size=2; lateral_secondary output size=2; axial_force_left input; grf_xz_left input; foot2com_x_left input; foot2com_z_left input; axial_force_secondary output; grf_xz_secondary output; foot2com_x_secondary output; foot2com_z_secondary output; x_state_secondary output; x_state_left input
% Switch between "primary" and "secondary" leg variables
function [leg_angle_primary, ...
          leg_length_primary, ...
          leg_width_primary, ...
          leg_roll_primary, ...
          back_load_primary, ...
          back_motor_primary, ...
          front_load_primary, ...
          front_motor_primary, ...
          lateral_primary, ...
          axial_force_primary, ...
          grf_xz_primary, ...
          foot2com_x_primary, ...
          foot2com_z_primary, ...
          x_state_primary, ...
          leg_angle_secondary, ...
          leg_length_secondary, ...
          leg_width_secondary, ...
          leg_roll_secondary, ...
          back_load_secondary, ...
          back_motor_secondary, ...
          front_load_secondary, ...
          front_motor_secondary, ...
          lateral_secondary, ...
          axial_force_secondary, ...
          grf_xz_secondary, ...
          foot2com_x_secondary, ...
          foot2com_z_secondary, ...
          x_state_secondary] ...
          = SignalSwitch(...
          right_is_primary, ...
          leg_angle_right, ...
          leg_length_right, ...
          leg_width_right, ...
          leg_roll_right, ...
          back_load_right, ...
          back_motor_right, ...
          front_load_right, ...
          front_motor_right, ...
          lateral_right, ...
          axial_force_right, ...
          grf_xz_right, ...
          foot2com_x_right, ...
          foot2com_z_right, ...
          x_state_right, ...
          leg_angle_left, ...
          leg_length_left, ...
          leg_width_left, ...
          leg_roll_left, ...
          back_load_left, ...
          back_motor_left, ...
          front_load_left, ...
          front_motor_left, ...
          lateral_left, ...
          axial_force_left, ...
          grf_xz_left, ...
          foot2com_x_left, ...
          foot2com_z_left, ...
          x_state_left)

if right_is_primary % right leg is primary
  leg_angle_primary = leg_angle_right;
  leg_length_primary = leg_length_right;
  leg_width_primary = leg_width_right;
  leg_roll_primary = leg_roll_right;
  back_load_primary = back_load_right;
  back_motor_primary = back_motor_right;
  front_load_primary = front_load_right;
  front_motor_primary = front_motor_right;
  lateral_primary = lateral_right;
  axial_force_primary = axial_force_right;
  grf_xz_primary = grf_xz_right;
  foot2com_x_primary = foot2com_x_right;
  foot2com_z_primary = foot2com_z_right;
  x_state_primary = x_state_right;
  leg_angle_secondary = leg_angle_left;
  leg_length_secondary = leg_length_left;
  leg_width_secondary = leg_width_left;
  leg_roll_secondary = leg_roll_left;
  back_load_secondary = back_load_left;
  back_motor_secondary = back_motor_left;
  front_load_secondary = front_load_left;
  front_motor_secondary = front_motor_left;
  lateral_secondary = lateral_left;
  axial_force_secondary = axial_force_left;
  grf_xz_secondary = grf_xz_left;
  foot2com_x_secondary = foot2com_x_left;
  foot2com_z_secondary = foot2com_z_left;
  x_state_secondary = x_state_left;
else % left leg is primary
  leg_angle_primary = leg_angle_left;
  leg_length_primary = leg_length_left;
  leg_width_primary = leg_width_left;
  leg_roll_primary = leg_roll_left;
  back_load_primary = back_load_left;
  back_motor_primary = back_motor_left;
  front_load_primary = front_load_left;
  front_motor_primary = front_motor_left;
  lateral_primary = lateral_left;
  axial_force_primary = axial_force_left;
  grf_xz_primary = grf_xz_left;
  foot2com_x_primary = foot2com_x_left;
  foot2com_z_primary = foot2com_z_left;
  x_state_primary = x_state_left;
  leg_angle_secondary = leg_angle_right;
  leg_length_secondary = leg_length_right;
  leg_width_secondary = leg_width_right;
  leg_roll_secondary = leg_roll_right;
  back_load_secondary = back_load_right;
  back_motor_secondary = back_motor_right;
  front_load_secondary = front_load_right;
  front_motor_secondary = front_motor_right;
  lateral_secondary = lateral_right;
  axial_force_secondary = axial_force_right;
  grf_xz_secondary = grf_xz_right;
  foot2com_x_secondary = foot2com_x_right;
  foot2com_z_secondary = foot2com_z_right;
  x_state_secondary = x_state_right;
end
